simulink model "ExerciseModel_18072025"  (R2025a)
settings: Solver=ode4  StartTime=0.0  StopTime=tsim  FixedStep=1  RelTol=1e-3
model workspace (MAT data in the model file):
  step_size = 1
values from neighbouring files (symbols this model uses):
  A_w = [cosd(beta1)*sind(alfa1)  -cosd(beta2)*sind(alfa2) -cosd(beta3)*sind(alfa3) cosd(beta4)*sind(alfa4) ... (first row only)    [initfun_18072025.m]    (also in initfun_18072025_nogyro.m)
  A_wP = pinv(A_w)    [initfun_18072025.m]    (also in initfun_18072025_nogyro.m)
  ARW = deg2rad(0.23)/sqrt(3600)    [initfun_18072025.m]
  Bias = deg2rad(1)/3600    [initfun_18072025.m]
  C_d = 2.2    [initfun_18072025.m]    (also in initfun_18072025_nogyro.m)
  d_max = 0.29    [initfun_18072025.m]    (also in initfun_18072025_nogyro.m)
  d_min = 0    [initfun_18072025.m]    (also in initfun_18072025_nogyro.m)
  ET0 = cspice_str2et(Date_UTC)    [initfun_18072025.m]    (also in initfun_18072025_nogyro.m)
  FOV = 166    [initfun_18072025.m]    (also in initfun_18072025_nogyro.m)
  G_earth = 6.6742e-11    [initfun_18072025.m]    (also in initfun_18072025_nogyro.m)
  init_state = [initial_position,initial_velocity,ang_vel_init2,quat_0]'    [initfun_18072025.m]    (also in initfun_18072025_nogyro.m)
  K = [F Z(:); Z(:)' sigma]    [Gain_matrix.m]    (also in QUEST.m = Gain_matrix(V',W',a); initfun_18072025.m = schmidt(nmax, mmax); initfun_18072025_nogyro.m = schmidt(nmax, mmax))
  K_dp = K_d_pitch_1    [evaluate_gains.m]    (also in evaluate_gains_nogyro.m)
  K_dr = K_d_roll_1    [evaluate_gains.m]    (also in evaluate_gains_nogyro.m)
  K_dy = K_d_yaw_1    [evaluate_gains.m]    (also in evaluate_gains_nogyro.m)
  K_pp = K_p_pitch_1    [evaluate_gains.m]    (also in evaluate_gains_nogyro.m; initfun_18072025_nogyro.m = K_pp/2)
  K_pr = K_p_roll_1    [evaluate_gains.m]    (also in evaluate_gains_nogyro.m; initfun_18072025.m = K_pr*1.8)
  K_py = K_p_yaw_1    [evaluate_gains.m]    (also in evaluate_gains_nogyro.m; initfun_18072025.m = K_py*10)
  m_earth = 5.9736e24    (= 5.9736e+24)    [initfun_18072025.m]    (also in initfun_18072025_nogyro.m)
  Magnetic_dipole = [0.1; 0.1;  0.1]    [initfun_18072025.m]    (also in initfun_18072025_nogyro.m)
  Magnetometers_number = 2    [initfun_18072025.m]    (also in initfun_18072025_nogyro.m)
  Mean_cart_Mag = 0    [initfun_18072025.m]    (also in initfun_18072025_nogyro.m)
  MeanangularSun = 0    [initfun_18072025.m]    (also in initfun_18072025_nogyro.m)
  mmax = 3    [initfun_18072025.m]    (also in initfun_18072025_nogyro.m)
  nmax = 3    [initfun_18072025.m]    (also in initfun_18072025_nogyro.m)
  omegaOrb = [0;-2*pi/P;0]    [initfun_18072025.m]    (also in initfun_18072025_nogyro.m)
  P_prev = [P_dg, zeros(3,3) ... (first row only)    [initfun_18072025.m]    (also in initfun_18072025_nogyro.m)
  P_sun = 4.56e-6    (= 4.56e-06)    [initfun_18072025.m]    (also in initfun_18072025_nogyro.m)
  Q = [eye(3,3).*Qattitudefactor zeros(3,3) ... (first row only)    [initfun_18072025.m]    (also in initfun_18072025_nogyro.m)
  R_B = (Sigma_cart_Mag)^2    (= 2.77777777778e-16)    [initfun_18072025.m]    (also in initfun_18072025_nogyro.m)
  r_earth = 6371e3    (= 6371000)    [initfun_18072025.m]    (also in initfun_18072025_nogyro.m)
  R_G = ARW^2    [initfun_18072025.m]
  R_SS = (SigmaangularSun*pi/180)^2    (= 3.04617419787e-06)    [initfun_18072025.m]    (also in initfun_18072025_nogyro.m)
  RWs_Inertia = diag([9.0718e-06, 9.0718e-06, 9.0718e-06, 9.0718e-06])    [initfun_18072025.m]    (also in initfun_18072025_nogyro.m)
  RWs_Inertia_Inv = inv(RWs_Inertia)    [initfun_18072025.m]    (also in initfun_18072025_nogyro.m)
  Sat_Inertia = diag([6.295, 1.644, 5.462]*10^-1)    [initfun_18072025.m]    (also in initfun_18072025_nogyro.m)
  Sat_mass = 12.172    [initfun_18072025.m]    (also in initfun_18072025_nogyro.m)
  Sigma_cart_Mag = (50*10^-9)/3    (= 1.66666666667e-08)    [initfun_18072025.m]    (also in initfun_18072025_nogyro.m)
  SigmaangularSun = 0.1    [initfun_18072025.m]    (also in initfun_18072025_nogyro.m)
  Sun_sensors = zeros(3, SS_number)    [initfun_18072025.m]    (also in initfun_18072025_nogyro.m)
  threshold_omega = omega_max * 0.8    (= 837.7580408)    [initfun_18072025.m]    (also in initfun_18072025_nogyro.m)
  x_prev = x0    [initfun_18072025.m]    (also in initfun_18072025_nogyro.m)
undefined symbols (not defined in the file or in its folder): DiscIntNeverNeededParam, G, H, IAU, juliandate, quat_feed_reg, Sat_Aeromodel_det
libraries: matrix_library x9, vrlib x2, aerolibtransform2 x1
(part 3 of 3)

== matlab function ExerciseModel_18072025/Spacecraft Dynamics Model/Equations of motion of the spacecraft ==
  data: f input; drag input; m input; I input; h_w input; T_control input; dfdt output; T_ext input
function dfdt = SpacecraftDynamicsSimulator(f, drag, m,I,h_w, T_control, T_ext)
%#codegen
%% Copyright Università di Napoli "Federico II" - Tutti i diritti sono riservati
%
% This function calculates the spacecraft acceleration from its
% position and velocity at time t.
%----------------------------------------------------------------------
mu = 398600; %Gravitational parameter (km^3/s^2)
RE = 6371; %Earth's radius (km)

x = f(1);    %Position vector component 1st axis (km)
y = f(2);    %Position vector component 2nd axis (km)
z = f(3);    %Position vector component 3rd axis (km)

R = f(1:3)'; %Position vector (km)
r = norm(R); %Distance from earth's center (km)

V = f(4:6);   %Velocity vector in ECI (km/s);

% Gravitational Perturbations Coefficients

J2 = 0.00108263;
J3 = -2.33936e-3*J2;
J4 = -1.49601e-3*J2;

% Central Body Keplerian Gravity
a0 = -mu*R/r^3; %Gravitational acceleration (km/s^2)

% Gravitational perturbation acceleration
a_J2 = 3*J2*mu*RE^2/2*...
    [x*5*z^2*(x^2+y^2+z^2)^(-7/2) - x*(x^2+y^2+z^2)^(-5/2),...
    y*5*z^2*(x^2+y^2+z^2)^(-7/2) - y*(x^2+y^2+z^2)^(-5/2),...
    5*z^3*(x^2+y^2+z^2)^(-7/2) - 3*z*(x^2+y^2+z^2)^(-5/2)];

a_J3 = 5*J3*mu*RE^3/2*...
    [-3*x*z*(x^2+y^2+z^2)^(-7/2) + 7*x*z^3*(x^2+y^2+z^2)^(-9/2),...
    -3*y*z*(x^2+y^2+z^2)^(-7/2) + 7*y*z^3*(x^2+y^2+z^2)^(-9/2),...
    3/5*(x^2+y^2+z^2)^(-5/2) - 6*z^2*(x^2+y^2+z^2)^(-7/2) + 7*z^4*(x^2+y^2+z^2)^(-9/2)];
a_J4 = 15*J4*mu*RE^4/8*...
    [x*(x^2+y^2+z^2)^(-7/2) - 14*x*z^2*(x^2+y^2+z^2)^(-9/2) + 21*x*z^4*(x^2+y^2+z^2)^(-11/2),...
    y*(x^2+y^2+z^2)^(-7/2) - 14*y*z^2*(x^2+y^2+z^2)^(-9/2) + 21*y*z^4*(x^2+y^2+z^2)^(-11/2),...
    5*z*(x^2+y^2+z^2)^(-7/2) - 70/3*z^3*(x^2+y^2+z^2)^(-9/2) + 21*z^5*(x^2+y^2+z^2)^(-11/2)];

% Translational Propagation equation (i.e. translational dynamic model)
a = a0' - drag*(1/m)*(1/1000) + a_J2' + a_J3' + a_J4'; %Total acceleration (km/s^2)

%% Rotational Dynamics;
w = f(7:9);       %Angular Velocity after the integration;

p = w(1);         %Angular Velocity component in BRF wrt ECI (1st axis)
q = w(2);         %Angular Velocity component in BRF wrt ECI (2nd axis)
r = w(3);         %Angular Velocity component in BRF wrt ECI (3rd axis)

J=inv(I);          %inverse inertia matrix;
h=I*w;             %angular momentum of the spacecraft;
A=cross(w,h+h_w);  %cross product;

w_dot=J*(T_ext-T_control-A); % Angular velocity rate of the body in BRF wrt ECI reference frame

   
%% Quaternions kynematics
q0 = f(10:13) / norm(f(10:13));                   %quaternion components (slide 5 of presentation lesson 2)
skew_mat = -[0 -w(3) w(2)        %Skew matrix for angular velocity quaternion multiplication (slide 5 of presentation lesson 2)  
            w(3) 0 -w(1)
           -w(2) w(1) 0];

q_dot_vec = 0.5*skew_mat*q0(1:3)+0.5*q0(4)*w;   %quaternion kinematics rate for propagation
q_dot_4 = -0.5*w'*q0(1:3);
q_dot = [q_dot_vec',q_dot_4]';                  %recollecting
%% Outputs
 
P = 2*pi*sqrt(6990^3/mu);
omegaOrb = [0;-2*pi/P;0];
dfdt = [V;a;w_dot;q_dot]; %Velocity and the acceleraion returned to ode45
%ciccio_caputo =1;
end
